simulink model "ModeWakeupManager"  (R2024a)
settings: Solver=VariableStepAuto  StartTime=0.0  StopTime=10.0  RelTol=1e-3
settings Model: DataDictionary=BMS_System_Arch_dict.sldd  Creator=ghourabi  LastModifiedBy=ghourabi

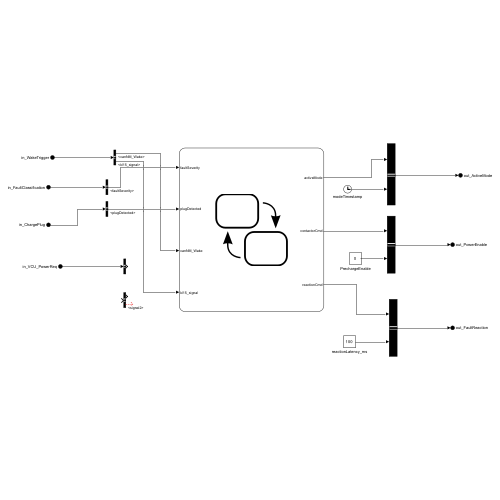
[thumbnail: Simulink's stored preview of the top-level diagram]
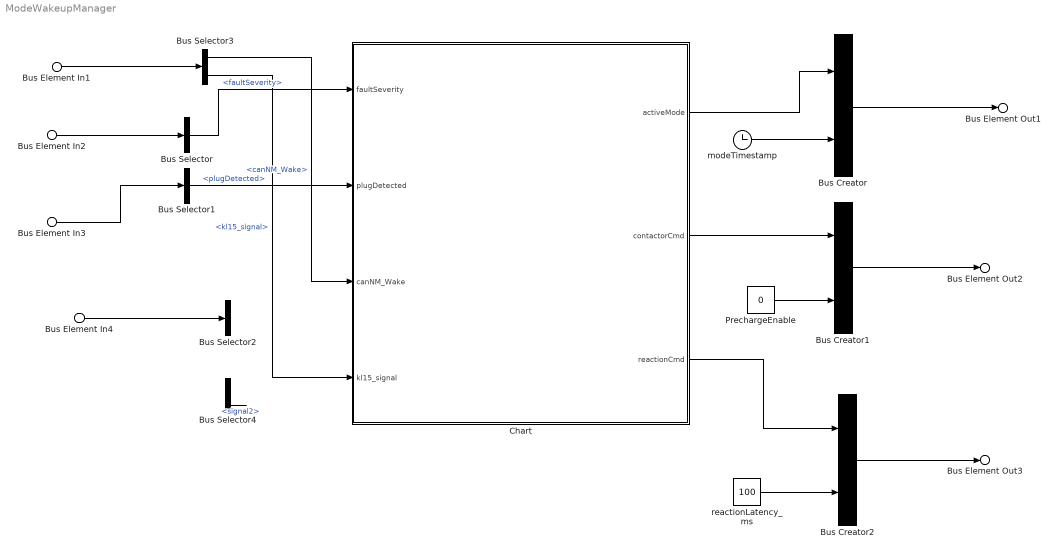
== system ModeWakeupManager ==
  Bus Element In1 : Inport  PortName=in_WakeTrigger
  Bus Element In2 : Inport  Port=2  PortName=in_FaultClassification
  Bus Element In3 : Inport  Port=3  PortName=in_ChargePlug
  Bus Element In4 : Inport  Port=4  PortName=in_VCU_PowerReq
  Bus Creator : BusCreator  Inputs=2
  Bus Creator1 : BusCreator  Inputs=2
  Bus Creator2 : BusCreator  Inputs=2
  Bus Selector : BusSelector  OutputSignals=faultSeverity
  Bus Selector1 : BusSelector  OutputSignals=plugDetected
  Bus Selector2 : BusSelector  OutputSignals=powerRequest_kW
  Bus Selector3 : BusSelector  OutputSignals=canNM_Wake,kl15_signal
  Bus Selector4 : BusSelector  OutputSignals=signal1,signal2
  Chart : Stateflow chart  TreatAsAtomicUnit=on
  PrechargeEnable : Constant  Value=0
  modeTimestamp : Clock
  reactionLatency_ms : Constant  Value=100
  Bus Element Out1 : Outport  PortName=out_ActiveMode
  Bus Element Out2 : Outport  Port=2  PortName=out_PowerEnable
  Bus Element Out3 : Outport  Port=3  PortName=out_FaultReaction
  wires:
  Bus Selector4/2 -> ?  "<signal2>"
  Bus Element In1/1 -> Bus Selector3/1
  Bus Element In2/1 -> Bus Selector/1
  Bus Element In3/1 -> Bus Selector1/1
  Bus Element In4/1 -> Bus Selector2/1
  Bus Selector/1 -> Chart/1(faultSeverity)  "<faultSeverity>"
  Bus Selector1/1 -> Chart/2(plugDetected)  "<plugDetected>"
  Bus Selector3/1 -> Chart/3(canNM_Wake)  "<canNM_Wake>"
  Bus Selector3/2 -> Chart/4(kl15_signal)  "<kl15_signal>"
  Chart/1(activeMode) -> Bus Creator/1
  modeTimestamp/1 -> Bus Creator/2
  Bus Creator/1 -> Bus Element Out1/1
  PrechargeEnable/1 -> Bus Creator1/2
  Bus Creator1/1 -> Bus Element Out2/1
  Chart/2(contactorCmd) -> Bus Creator1/1
  Chart/3(reactionCmd) -> Bus Creator2/1
  reactionLatency_ms/1 -> Bus Creator2/2
  Bus Creator2/1 -> Bus Element Out3/1

== stateflow chart ModeWakeupManager/Chart ==
  state INIT
    entry: activeMode = 0;
    contactorCmd = false;
    reactionCmd = 0;
  state CHARGING
    entry_ activeMode = 2;
    contactorCmd = true;
    reactionCmd = 0;
  state NORMAL
    entry: activeMode = 1;
    contactorCmd = true;
    reactionCmd = 0;
  state SLEEP
    entry_ activeMode = 5;
    contactorCmd = false;
    reactionCmd = 0;
  state LIMP
    entry: activeMode = 3;
    contactorCmd = true;
    reactionCmd = 1;
  state SAFE_STATE
    entry: activeMode = 4;
    contactorCmd = false;
    reactionCmd = 2;
  SLEEP -> INIT : [canNM_Wake == true || kl15_signal == true]
  (default) -> INIT [order 1]
  (default) -> CHARGING [order 3]
  SAFE_STATE -> INIT : [after(5, sec)]
      |   (reset après 5s — simplifié)
  INIT -> NORMAL : [[after(0.5, sec)]]
  NORMAL -> CHARGING [order 1] : [plugDetected == true]
  (default) -> NORMAL [order 2]
  CHARGING -> NORMAL : [plugDetected == false]
  NORMAL -> LIMP [order 2] : [faultSeverity == 1]
  NORMAL -> SAFE_STATE [order 3] : [faultSeverity == 2]
  NORMAL -> SLEEP [order 4] : [kl15_signal == false]
  (default) -> SLEEP [order 6]
  (default) -> LIMP [order 4]
  (default) -> SAFE_STATE [order 5]
  LIMP -> SAFE_STATE : [faultSeverity == 2]
  data: faultSeverity input int32; plugDetected input boolean; canNM_Wake input boolean; kl15_signal input boolean; activeMode output int32 =0; contactorCmd output boolean =false; reactionCmd output int32 =0
